simulink model "ModeloMIMO"  (R2022a)
settings: Solver=VariableStepAuto  StartTime=0.0  StopTime=300  FixedStep=0.279098492389953  RelTol=1e-3
model workspace (MAT data in the model file):
  ca = 0.02
  cb = 0.2
  ea = 0.06
  eb = 0.02
  pa = 3
  pb = 3
  u = 0.07
  v = 4
undefined symbols (not defined in the file or in its folder): sigbuilder_block
settings Model: Creator=Asus  LastModifiedBy=Abelino
settings DataIOCC: SaveFormat=Array  OutputTimes=tout

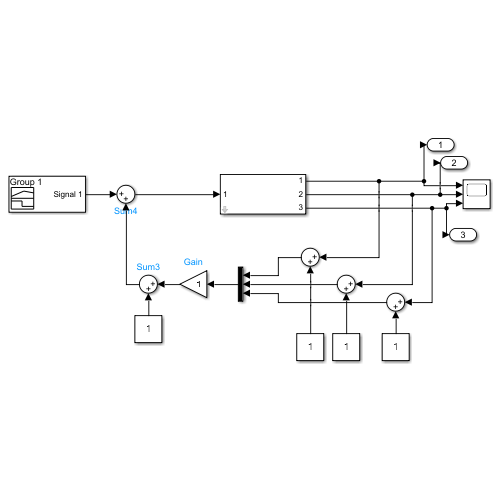
[thumbnail: Simulink's stored preview of the top-level diagram]
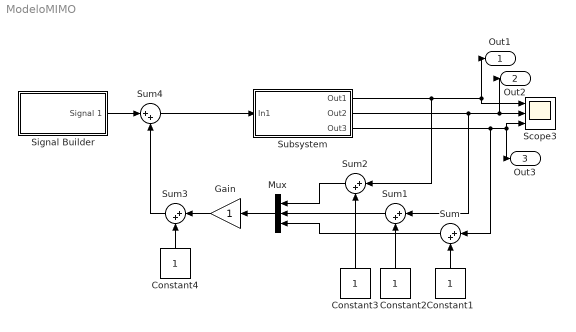
== system ModeloMIMO ==
  Constant{1..4} (4 alike) : Constant
  Gain : Gain
  Mux : Mux  Inputs=3
  Scope3 : Scope  NumInputPorts=3
  Signal Builder : Subsystem  Tag=STV Subsys  LoadFcn=sigbuilder_block('load');  StartFcn=sigbuilder_block('start');  StopFcn=sigbuilder_block('stop');  ClipboardFcn=sigbuilder_block('clipboard');  mask(Sigbuilder block){tuvar=[0:10]}
      mask help: Simulink:masks:SigbuilderBlock_MD
      mask init:
      | if ~strcmp(get_param(bdroot(gcbh),'SimulationStatus'),'stopped') tuvar = sigbuilder_block('maskInit'); end
      settings: CopyFcn=sigbuilder_block('copy');  DeleteFcn=sigbuilder_block('delete');  ModelCloseFcn=sigbuilder_block('modelClose');  PreSaveFcn=sigbuilder_block('preSave');  PauseFcn=sigbuilder_block('pause');  ContinueFcn=sigbuilder_block('continue');  NameChangeFcn=sigbuilder_block('namechange');  OpenFcn=sigbuilder_block('open',[437.6 199.2 550.4 400 ]);  CloseFcn=sigbuilder_block('close');
      mask Display: plot(0, 0, 100, 100,[2, 2, 32, 32, 2], [68, 8, 8, 68, 68],[32, 2], [38, 38], [32, 19, 2],[53, 60, 44], [32, 17, 17, 2],[16, 16, 31, 31]);txt = getActiveGroup(gcbh);text(2, 100, txt,'verticalAlignment', 'top');
  Subsystem : Subsystem  mask{ea=ea, eb=eb, ca=ca, cb=cb, pa=pa, pb=pb, v=v}
      mask prompts: ea "Tasa de extinción competidor A"; eb "Tasa de extinción del competidor B"; ca "Tasa de colonización del competidor A"; cb "Tasa de colonización del competidor B"; pa "Condición inicial x1"; pb "Condicion inicial x2"; v "Condicion inicial x3"
  Sum{,1..4} (5 alike) : Sum  Inputs=|++
  Out1 : Outport
  Out2 : Outport  Port=2
  Out3 : Outport  Port=3
  wires:
  Subsystem/2(Out2) -> Out2/1, Scope3/2, Sum1/1
  Subsystem/3(Out3) -> Sum/1, Scope3/3, Out3/1
  Subsystem/1(Out1) -> Scope3/1, Out1/1, Sum2/1
  Sum4/1 -> Subsystem/1(In1)
  Constant1/1 -> Sum/2
  Constant2/1 -> Sum1/2
  Constant3/1 -> Sum2/2
  Sum2/1 -> Mux/1
  Sum1/1 -> Mux/2
  Sum/1 -> Mux/3
  Mux/1 -> Gain/1
  Gain/1 -> Sum3/1
  Constant4/1 -> Sum3/2
  Sum3/1 -> Sum4/2
  Signal Builder/1(Signal 1) -> Sum4/1

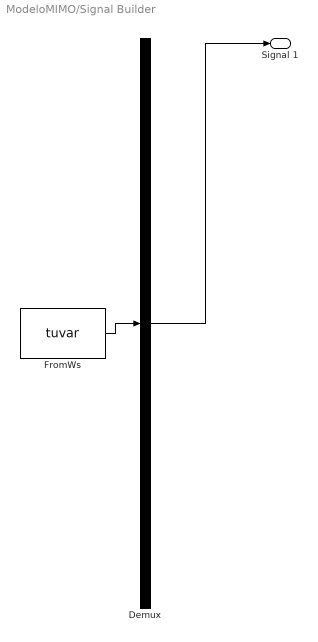
== system ModeloMIMO/Signal Builder ==
  Demux : Demux  Tag=STV Demux  Outputs=1
      settings: DisplayOption=none
  FromWs : FromWorkspace  Tag=STV FromWs  VariableName=tuvar
      SigBuilderData=|
      | common.afterFinalStr = 'Extrapolate'
      | common.sampleTime = 0
      | dataSet.timeRange = [0 10]
      | dataSet.name = 'Group 1'
      | sbobj.Groups.Name = 'Group 1'
      | sbobj.Groups.Signals.Name = 'Signal 1'
      | sbobj.Groups.Signals.XData = [0 4 4 6 6 10]
      | sbobj.Groups.Signals.YData = [0 0 1 1 0 0]
  Signal 1 : Outport  Tag=STV Outport
  wires:
  Demux/1 -> Signal 1/1
  FromWs/1 -> Demux/1

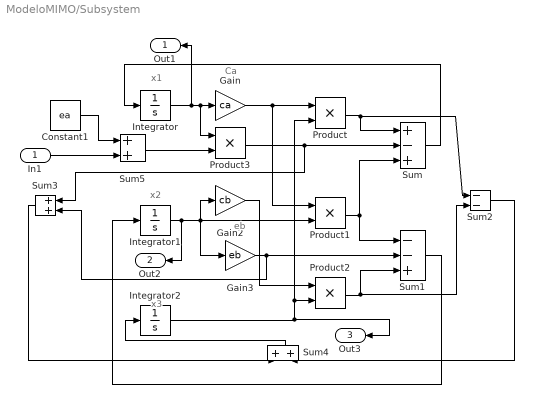
== system ModeloMIMO/Subsystem ==
  note: x1
  note: x3
  note: x2
  note: eb
  note: Ca
  In1 : Inport
  Constant1 : Constant  Value=ea
  Gain : Gain  Gain=ca
  Gain2 : Gain  Gain=cb
  Gain3 : Gain  Gain=eb
  Integrator : Integrator  InitialCondition=pa  LimitOutput=on  LowerSaturationLimit=0
  Integrator1 : Integrator  InitialCondition=pb  LimitOutput=on  LowerSaturationLimit=0
  Integrator2 : Integrator  InitialCondition=v  LimitOutput=on  LowerSaturationLimit=0
  Product{,1..3} (4 alike) : Product
  Sum : Sum  Inputs=+-+
  Sum1 : Sum  Inputs=--+
  Sum2 : Sum  Inputs=--
  Sum3 : Sum
  Sum4 : Sum
  Sum5 : Sum
  Out1 : Outport
  Out2 : Outport  Port=2
  Out3 : Outport  Port=3
  wires:
  Integrator/1 -> Out1/1, Product3/1, Gain/1
  Gain/1 -> Product1/1, Product/1
  Integrator2/1 -> Product/2, Product2/2, Out3/1
  Sum4/1 -> Integrator2/1
  Product2/1 -> Sum2/2, Sum1/3
  Sum2/1 -> Sum4/2
  Product/1 -> Sum2/1, Sum/1
  Gain2/1 -> Product2/1
  Gain3/1 -> Sum3/2, Sum1/2
  Sum3/1 -> Sum4/1
  Integrator1/1 -> Out2/1, Gain3/1, Gain2/1, Product1/2
  Sum/1 -> Integrator/1
  Product1/1 -> Sum/3, Sum1/1
  Sum1/1 -> Integrator1/1
  Constant1/1 -> Sum5/1
  In1/1 -> Sum5/2
  Sum5/1 -> Product3/2
  Product3/1 -> Sum3/1, Sum/2
